simulink model "lab7task"  (R2018a)
settings: Solver=VariableStepAuto  StartTime=0.0  StopTime=1  RelTol=1e-3
libraries: dsparch4 x1
settings Model: Creator=symih  LastModifiedBy=symih

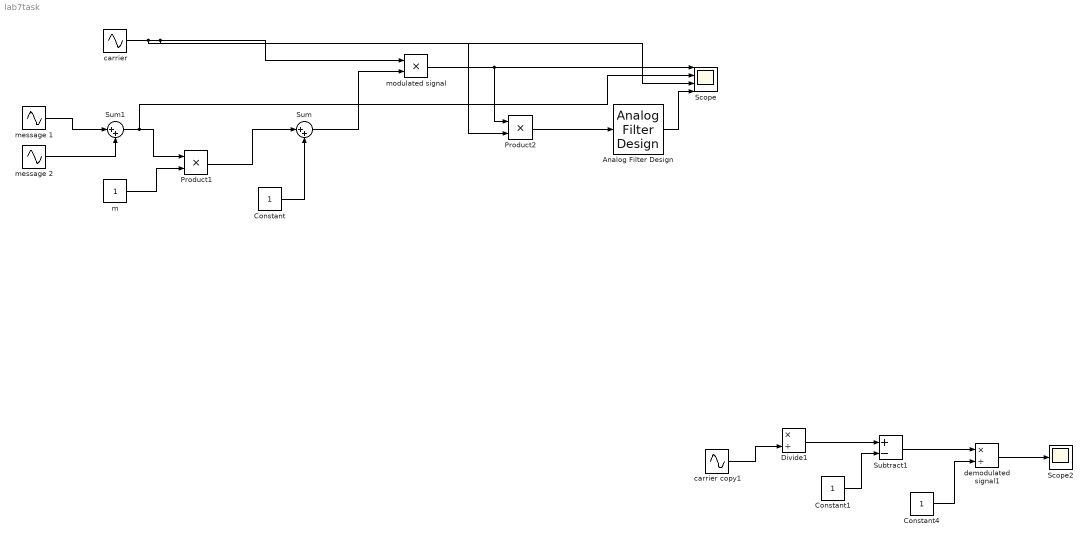
== system lab7task ==
  Analog Filter Design : dsparch4/Analog Filter Design  method=Butterworth  filttype=Lowpass  N=8  Wlo=30  Whi=80  Rp=2  Rs=40
  Constant : Constant
  Constant1 : Constant
  Constant4 : Constant
  Divide1 : Product  Inputs=*/
  Product1 : Product
  Product2 : Product
  Scope : Scope  NumInputPorts=4
  Scope2 : Scope
  Subtract1 : Sum  Inputs=+-
  Sum : Sum  Inputs=|++
  Sum1 : Sum  Inputs=|++
  carrier : Sin  Frequency=2*pi*50  Phase=pi/2  SampleTime=0
  carrier copy1 : Sin  Frequency=2*pi*50  Phase=pi/2  SampleTime=0
  demodulated signal1 : Product  Inputs=*/
  m : Constant
  message 1 : Sin  Frequency=2*pi*4  SampleTime=0
  message 2 : Sin  Frequency=2*pi*6  Phase=pi/2  SampleTime=0
  modulated signal : Product
  wires:
  message 1/1 -> Sum1/1
  message 2/1 -> Sum1/2
  m/1 -> Product1/2
  Constant/1 -> Sum/2
  Product1/1 -> Sum/1
  Sum/1 -> modulated signal/2
  modulated signal/1 -> Product2/1, Scope/1
  Sum1/1 -> Scope/2, Product1/1
  carrier/1 -> Product2/2, Scope/3, modulated signal/1
  Divide1/1 -> Subtract1/1
  Constant4/1 -> demodulated signal1/2
  Constant1/1 -> Subtract1/2
  Subtract1/1 -> demodulated signal1/1
  demodulated signal1/1 -> Scope2/1
  carrier copy1/1 -> Divide1/2
  Analog Filter Design/1 -> Scope/4
  Product2/1 -> Analog Filter Design/1
